simulink model "driver_simulink"  (R2013a)
settings: Solver=ode45  StartTime=0.0  StopTime=10.0  RelTol=1e-3
values from neighbouring files (symbols this model uses):
  TauSW = 18    [data_driver.m]
undefined symbols (not defined in the file or in its folder): driver, traiettoria
libraries: simulink x1
settings Model: Creator=ebertocchi  LastModifiedBy=ebertocchi

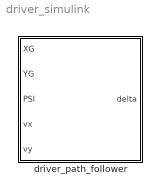
== system driver_simulink ==
  driver_path_follower : Subsystem

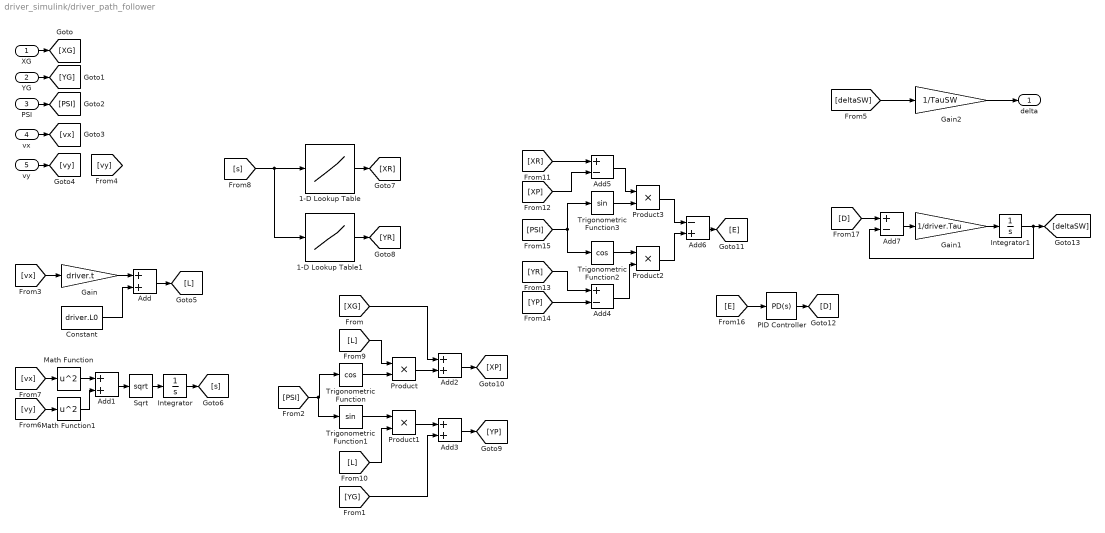
== system driver_simulink/driver_path_follower ==
  XG : Inport
  YG : Inport  Port=2
  PSI : Inport  Port=3
  vx : Inport  Port=4
  vy : Inport  Port=5
  1-D Lookup Table : Lookup_n-D  NumberOfTableDimensions=1  BreakpointsForDimension1=traiettoria.s  BeginIndexSearchUsingPreviousIndexResult=on  Table=traiettoria.x  RndMeth=Simplest  InputSameDT=on
  1-D Lookup Table1 : Lookup_n-D  NumberOfTableDimensions=1  BreakpointsForDimension1=traiettoria.s  Table=traiettoria.y  RndMeth=Simplest  InputSameDT=on
  Add{,1..3} (4 alike) : Sum
  Add4 : Sum  Inputs=+-
  Add5 : Sum  Inputs=+-
  Add6 : Sum  Inputs=-+
  Add7 : Sum  Inputs=+-
  Constant : Constant  Value=driver.L0
  Gain : Gain  Gain=driver.t
  Gain1 : Gain  Gain=1/driver.Tau
  Gain2 : Gain  Gain=1/TauSW
  Integrator : Integrator
  Integrator1 : Integrator
  Math Function : Math  Operator=square  SaturateOnIntegerOverflow=on
  Math Function1 : Math  Operator=square  SaturateOnIntegerOverflow=on
  PID Controller : simulink/Continuous/PID Controller  Controller=PD  TimeDomain=Continuous-time  SampleTime=1  IntegratorMethod=Forward Euler  FilterMethod=Forward Euler  Form=Parallel  P=driver.kP  I=1  D=driver.kD  N=100  InitialConditionSource=internal  InitialConditionForIntegrator=0  InitialConditionForFilter=0  ExternalReset=none  LimitOutput=off  UpperSaturationLimit=inf  LowerSaturationLimit=-inf  LinearizeAsGain=on  AntiWindupMode=none  Kb=1  TrackingMode=off  Kt=1  PParamMin=[]  PParamMax=[]  IParamMin=[]  IParamMax=[]  DParamMin=[]  DParamMax=[]  NParamMin=[]  NParamMax=[]  KbParamMin=[]  KbParamMax=[]  KtParamMin=[]  KtParamMax=[]  POutMin=[]  POutMax=[]  IOutMin=[]  IOutMax=[]  DOutMin=[]  DOutMax=[]  NOutMin=[]  NOutMax=[]  KbOutMin=[]  KbOutMax=[]  KtOutMin=[]  KtOutMax=[]  IntegratorOutMin=[]  IntegratorOutMax=[]  FilterOutMin=[]  FilterOutMax=[]  SumOutMin=[]  SumOutMax=[]  SumI1OutMin=[]  SumI1OutMax=[]  SumI2OutMin=[]  SumI2OutMax=[]  SumI3OutMin=[]  SumI3OutMax=[]  SumDOutMin=[]  SumDOutMax=[]  SaturationOutMin=[]  SaturationOutMax=[]  IntegratorContinuousStateAttributes=''  IntegratorStateMustResolveToSignalObject=off  IntegratorRTWStateStorageClass=Auto  FilterContinuousStateAttributes=''  FilterStateMustResolveToSignalObject=off  FilterRTWStateStorageClass=Auto
  Product{,1..3} (4 alike) : Product
  Sqrt : Sqrt  SaturateOnIntegerOverflow=on
  Trigonometric Function : Trigonometry  Operator=cos
  Trigonometric Function1 : Trigonometry
  Trigonometric Function2 : Trigonometry  Operator=cos
  Trigonometric Function3 : Trigonometry
  delta : Outport
  wires:
  XG/1 -> [XG]
  YG/1 -> [YG]
  PSI/1 -> [PSI]
  vx/1 -> [vx]
  vy/1 -> [vy]
  [deltaSW] -> Gain2/1
  [vx] -> Gain/1
  Gain/1 -> Add/1
  Constant/1 -> Add/2
  Add/1 -> [L]
  [vx] -> Math Function/1
  [vy] -> Math Function1/1
  Math Function/1 -> Add1/1
  Math Function1/1 -> Add1/2
  Add1/1 -> Sqrt/1
  Sqrt/1 -> Integrator/1
  Integrator/1 -> [s]
  [s] -> 1-D Lookup Table1/1, 1-D Lookup Table/1
  1-D Lookup Table/1 -> [XR]
  1-D Lookup Table1/1 -> [YR]
  [PSI] -> Trigonometric Function1/1, Trigonometric Function/1
  Trigonometric Function/1 -> Product/2
  Trigonometric Function1/1 -> Product1/1
  [L] -> Product1/2
  [L] -> Product/1
  Product/1 -> Add2/2
  [XG] -> Add2/1
  Product1/1 -> Add3/1
  [YG] -> Add3/2
  Add3/1 -> [YP]
  Add2/1 -> [XP]
  [PSI] -> Trigonometric Function2/1, Trigonometric Function3/1
  [YP] -> Add4/2
  [YR] -> Add4/1
  [XR] -> Add5/1
  [XP] -> Add5/2
  Trigonometric Function2/1 -> Product2/1
  Add4/1 -> Product2/2
  Trigonometric Function3/1 -> Product3/2
  Add5/1 -> Product3/1
  Product3/1 -> Add6/1
  Product2/1 -> Add6/2
  Add6/1 -> [E]
  [E] -> PID Controller/1
  PID Controller/1 -> [D]
  [D] -> Add7/1
  Add7/1 -> Gain1/1
  Integrator1/1 -> Add7/2, [deltaSW]
  Gain1/1 -> Integrator1/1
  Gain2/1 -> delta/1
